simulink model "Ldg_1_gruppo_6_2024_2025_DIN_LONG"  (R2023b)
settings: Solver=ode4  StartTime=0.0  StopTime=10.0  FixedStep=0.1  RelTol=1e-3
values from neighbouring files (symbols this model uses):
  de0_air3m = U0_air3m(7)    [Ldg_1_gruppo_6_2024_2025.m]
  Fx0_air3m = U0_air3m(1)*10000    [Ldg_1_gruppo_6_2024_2025.m]
libraries: airlib x1
settings Model: Creator=Elisa  LastModifiedBy=Elisa

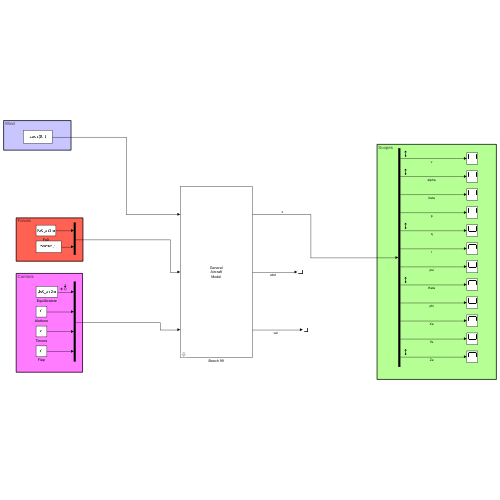
[thumbnail: Simulink's stored preview of the top-level diagram]
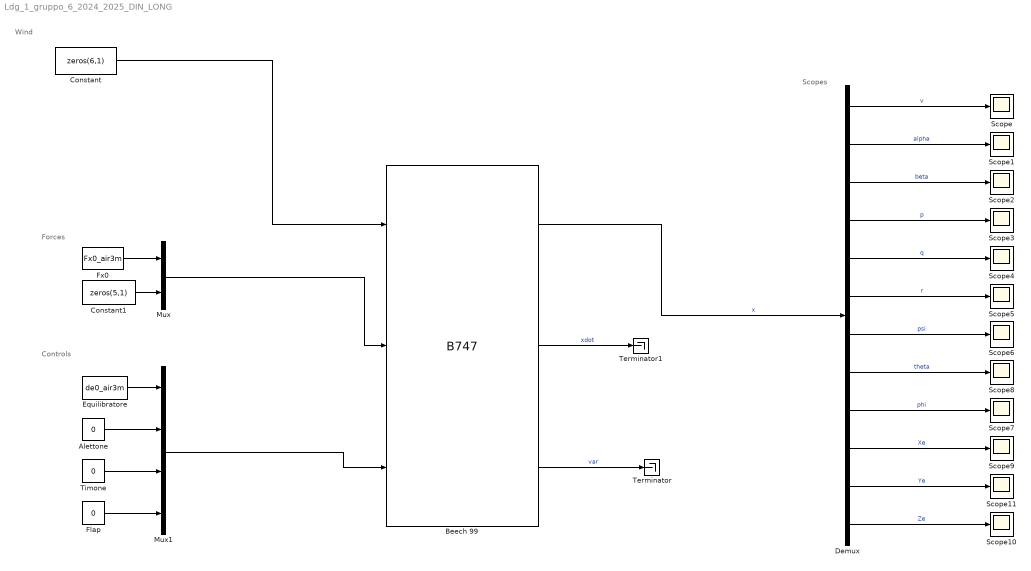
== system Ldg_1_gruppo_6_2024_2025_DIN_LONG ==
  note: Wind
  note: Controls
  note: Forces
  note: Scopes
  " Beech 99 " : airlib/B747  GM1="[1.9812   14.0208  26.0129  13673  20538  31246   0  2169.3  0   3175.2]"  CD_wind="[0.027   0.131  0  0  0]"  CL_wind="[0.201   5.48    8.1   0.6   0]"  Cm_body="[0.05  -1.89  -34.0   -2.0   0]"  CY_body="[0  -0.59  -0.19  0.39  0.0  0.148]"  Cl_body="[0    -0.13  -0.5  0.14  -0.156  0.0109]"  Cn_body="[0    0.08   0.0109  -0.197  0.0012  -0.0772]"  x0=X0_air3m
      settings: SourceProductName=Aircraft Library
  Alettone : Constant  Value=0
  Constant : Constant  Value=zeros(6,1)
  Constant1 : Constant  Value=zeros(5,1)
  Demux : Demux  Outputs=12
  Equilibratore : Constant  Value=de0_air3m
  Flap : Constant  Value=0
  Fx0 : Constant  Value=Fx0_air3m
  Mux : Mux  Inputs=2
  Mux1 : Mux
  Scope{,1..11} (12 alike) : Scope
  Terminator : Terminator
  Terminator1 : Terminator
  Timone : Constant  Value=0
  wires:
  Constant/1 -> " Beech 99 "/1
  " Beech 99 "/2 -> Terminator1/1  "xdot"
  " Beech 99 "/3 -> Terminator/1  "var"
  " Beech 99 "/1 -> Demux/1  "x"
  Mux/1 -> " Beech 99 "/2
  Demux/3 -> Scope2/1  "beta"
  Demux/8 -> Scope8/1  "theta"
  Demux/4 -> Scope3/1  "p"
  Demux/10 -> Scope9/1  "Xe"
  Demux/5 -> Scope4/1  "q"
  Equilibratore/1 -> Mux1/1
  Demux/6 -> Scope5/1  "r"
  Demux/12 -> Scope10/1  "Ze"
  Constant1/1 -> Mux/2
  Mux1/1 -> " Beech 99 "/3
  Flap/1 -> Mux1/4
  Demux/9 -> Scope7/1  "phi"
  Demux/7 -> Scope6/1  "psi"
  Demux/11 -> Scope11/1  "Ye"
  Alettone/1 -> Mux1/2
  Demux/2 -> Scope1/1  "alpha"
  Demux/1 -> Scope/1  "v"
  Timone/1 -> Mux1/3
  Fx0/1 -> Mux/1
